simulink model "Cell_Balancing"  (R2024a)
settings: Solver=FixedStepDiscrete  StartTime=0.0  StopTime=10.0  FixedStep=1e-3  RelTol=1e-3
settings Model: Creator=VICTUS  LastModifiedBy=VICTUS

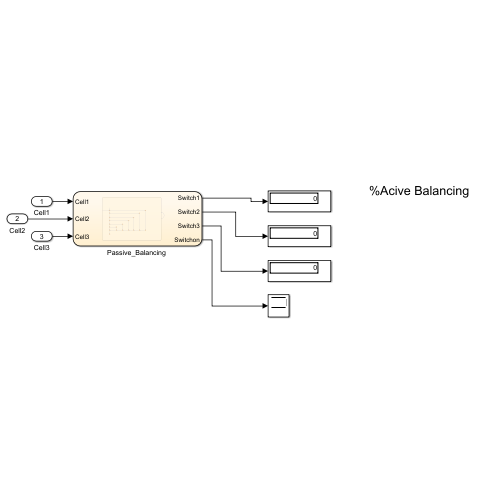
[thumbnail: Simulink's stored preview of the top-level diagram]
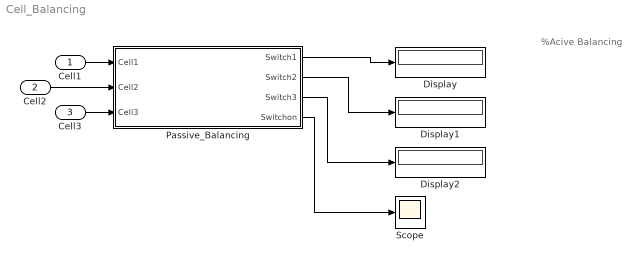
== system Cell_Balancing ==
  note: %Acive Balancing
  Cell1 : Inport
  Cell2 : Inport  Port=2
  Cell3 : Inport  Port=3
  Display : Display
  Display1 : Display
  Display2 : Display
  "Passive_Balancing " : Stateflow chart  TreatAsAtomicUnit=on
  Scope : Scope
  wires:
  "Passive_Balancing "/1(Switch1) -> Display/1
  "Passive_Balancing "/2(Switch2) -> Display1/1
  "Passive_Balancing "/3(Switch3) -> Display2/1
  Cell1/1 -> "Passive_Balancing "/1(Cell1)
  Cell2/1 -> "Passive_Balancing "/2(Cell2)
  Cell3/1 -> "Passive_Balancing "/3(Cell3)
  "Passive_Balancing "/4(Switchon) -> Scope/1

== stateflow chart Cell_Balancing/Passive_Balancing  ==
  state Passive_Balancing
    (default) -> (junction 16)
    Passive_Balancing -> (junction 16) [order 1]
    (junction 16) -> (junction 18) [order 1] : [Cell1 > Cell3  && Cell3 > Cell2]
    (junction 18) -> (junction 20) : {Switch1 = 1;Switch3 = 1;}
    (junction 16) -> (junction 24) [order 2]
    (junction 24) -> (junction 26) [order 1] : [Cell1 > Cell3  && Cell2 > Cell3]
    (junction 24) -> (junction 31) [order 2]
    (junction 26) -> (junction 28) : {Switch1 = 1;Switch2 = 1;}
    (junction 31) -> (junction 47) [order 1] : [Cell2 > Cell3  && Cell3 > Cell1]
    (junction 31) -> (junction 50) [order 2]
    (junction 47) -> (junction 54) : {Switch2 = 1;Switch3 = 1;}
    (junction 50) -> (junction 53) [order 1] : [Cell2 > Cell3  && Cell1 > Cell3]
    (junction 50) -> (junction 71) [order 2]
    (junction 53) -> (junction 52) : {Switch1 = 1;Switch2 = 1;}
    (junction 71) -> (junction 61) [order 1] : [Cell3 > Cell2  && Cell2 > Cell1]
    (junction 71) -> (junction 72) [order 2]
    (junction 61) -> (junction 70) : {Switch2 = 1;Switch3 = 1;}
    (junction 72) -> (junction 68) [order 1] : [Cell3 > Cell2  && Cell1 > Cell2]
    (junction 72) -> (junction 66) [order 2]
    (junction 68) -> (junction 67) : {Switch1 = 1;Switch3 = 1;}
    (junction 67) -> (junction 66)
    (junction 70) -> (junction 67)
    (junction 52) -> (junction 70)
    (junction 54) -> (junction 52)
    (junction 28) -> (junction 54)
    (junction 20) -> (junction 28)
    (junction 66) -> (junction 69)
  Passive_Balancing -> Passive_Balancing [order 1] : after(0.1,sec)/{Switchon}
  data: Cell1 input; Cell2 input; Cell3 input; Switch1 output; Switch2 output; Switch3 output
  events: Switchon output EITHER_EDGE_EVENT
